simulink model "SpaceXStarshipMotionSimulation"  (R2024b)
settings: Solver=VariableStepAuto  StartTime=0.0  StopTime=60  RelTol=1e-3
values from neighbouring files (symbols this model uses):
  c_p = 55.09    [SpaceX Starship_EarthtoEarth_Sims.m]
  F_t = 74400000    [SpaceX Starship_EarthtoEarth_Sims.m]
  g = 9.81    [SpaceX Starship_EarthtoEarth_Sims.m]
  Ixx = I(1,1)    [SpaceX Starship_EarthtoEarth_Sims.m]
  Izz = I(3,3)    [SpaceX Starship_EarthtoEarth_Sims.m]
  L = 55.74    [SpaceX Starship_EarthtoEarth_Sims.m]
  m_r = 5270000    [SpaceX Starship_EarthtoEarth_Sims.m]
libraries: simulink x9, shared6dof x1, aerolibanim x1
settings Model: Creator=samueljoseph  LastModifiedBy=samueljoseph

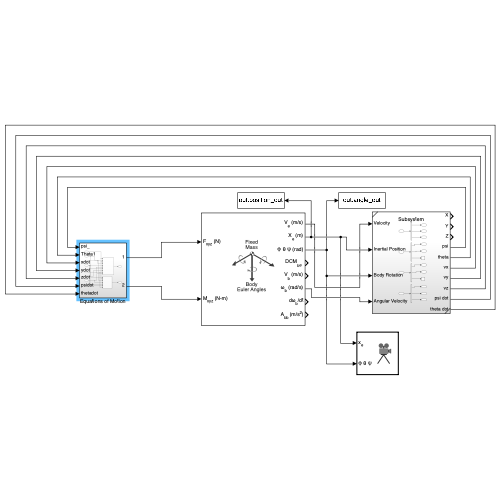
[thumbnail: Simulink's stored preview of the top-level diagram]
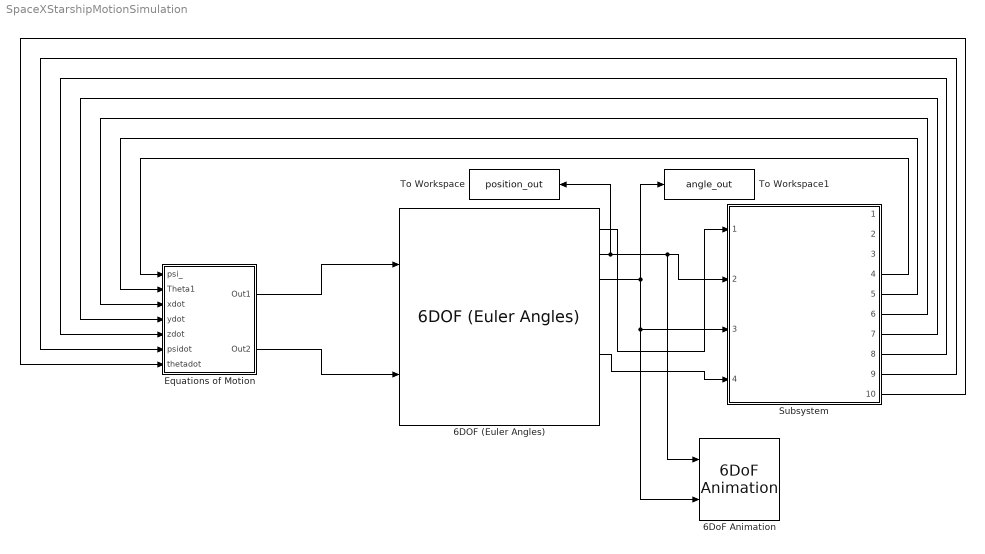
== system SpaceXStarshipMotionSimulation ==
  6DOF (Euler Angles) : shared6dof/6DOF (Euler Angles)  units=Metric (MKS)  mtype=Fixed  rep=Euler Angles  xme_0=[0 0 6371000]  Vm_0=[0 0 0]  eul_0=[pi/4 pi/4 0]  pm_0=[0 0 0]  mass_0=5270000  mass_e=0.5  mass_f=2.0  inertia=[1.9980e9 0 0; 0 1.9980e9 0; 0 0 13069836]  inertia_e=eye(3)  inertia_f=2*eye(3)  k_quat=1.0  vre_flag=on  abi_flag=off  aMode=0  xme_statename=''  Vm_statename=''  eul_statename=''  quat_statename=''  pm_statename=''  mass_statename=''
  6DoF Animation : aerolibanim/6DoF Animation  u1=[0 4000 -2000 2000 -20000 0]  u2=0.1  u3=2000  u4=[4000 0 -5000]  u5=Fly alongside  u6=[5000, 2000, 1000]  u7=45  u8=on
  Equations of Motion : Subsystem
  Subsystem : Subsystem  ReferencedSubsystem=Subsystem
  To Workspace : ToWorkspace  VariableName=position_out  SaveFormat=Timeseries  SampleTime=-1
  To Workspace1 : ToWorkspace  VariableName=angle_out  SaveFormat=Timeseries  SampleTime=-1
  wires:
  6DOF (Euler Angles)/6 -> Subsystem/4
  6DOF (Euler Angles)/2 -> 6DoF Animation/1, Subsystem/2, To Workspace/1
  6DOF (Euler Angles)/3 -> 6DoF Animation/2, Subsystem/3, To Workspace1/1
  6DOF (Euler Angles)/1 -> Subsystem/1
  Subsystem/4 -> Equations of Motion/1(psi_)
  Subsystem/5 -> Equations of Motion/2(Theta1)
  Subsystem/6 -> Equations of Motion/3(xdot)
  Subsystem/7 -> Equations of Motion/4(ydot)
  Subsystem/8 -> Equations of Motion/5(zdot)
  Subsystem/9 -> Equations of Motion/6(psidot)
  Subsystem/10 -> Equations of Motion/7(thetadot)
  Equations of Motion/1(Out1) -> 6DOF (Euler Angles)/1
  Equations of Motion/2(Out2) -> 6DOF (Euler Angles)/2

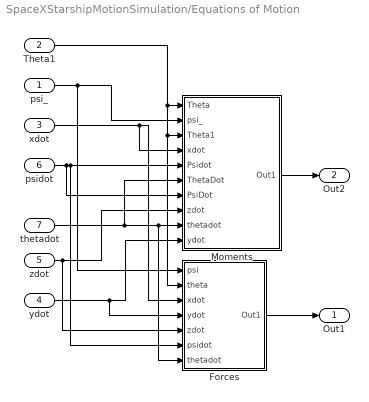
== system SpaceXStarshipMotionSimulation/Equations of Motion ==
  psi_ : Inport
  Theta1 : Inport  Port=2
  xdot : Inport  Port=3
  ydot : Inport  Port=4
  zdot : Inport  Port=5
  psidot : Inport  Port=6
  thetadot : Inport  Port=7
  Forces : Subsystem
  Moments : Subsystem
  Out1 : Outport
  Out2 : Outport  Port=2
  wires:
  Forces/1(Out1) -> Out1/1
  ydot/1 -> Moments/10(ydot), Forces/4(ydot)
  zdot/1 -> Moments/8(zdot), Forces/5(zdot)
  thetadot/1 -> Forces/7(thetadot), Moments/9(thetadot), Moments/6(ThetaDot)
  psidot/1 -> Moments/5(Psidot), Forces/6(psidot), Moments/7(PsiDot)
  xdot/1 -> Moments/4(xdot), Forces/3(xdot)
  Moments/1(Out1) -> Out2/1
  psi_/1 -> Moments/2(psi_), Forces/1(psi)
  Theta1/1 -> Forces/2(theta), Moments/3(Theta1), Moments/1(Theta)

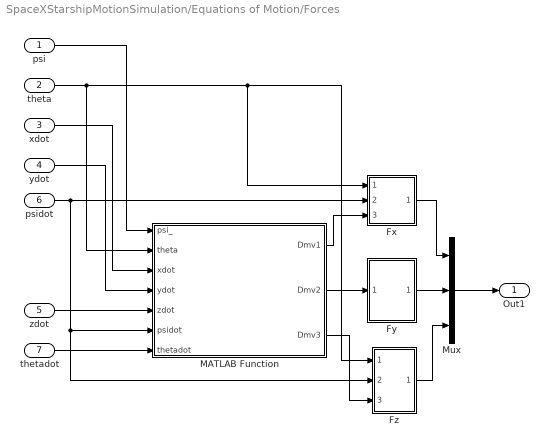
== system SpaceXStarshipMotionSimulation/Equations of Motion/Forces ==
  psi : Inport
  theta : Inport  Port=2
  xdot : Inport  Port=3
  ydot : Inport  Port=4
  zdot : Inport  Port=5
  psidot : Inport  Port=6
  thetadot : Inport  Port=7
  Fx : Subsystem
  Fy : Subsystem
  Fz : Subsystem
  MATLAB Function : MATLAB Function  TreatAsAtomicUnit=on
  Mux : Mux  Inputs=3
  Out1 : Outport
  wires:
  Mux/1 -> Out1/1
  Fz/1(Out1) -> Mux/3
  Fy/1(Out1) -> Mux/2
  Fx/1(Out1) -> Mux/1
  xdot/1 -> MATLAB Function/3(xdot)
  MATLAB Function/3(Dmv3) -> Fz/3(Dmv3)
  psidot/1 -> MATLAB Function/6(psidot), Fz/2(psidot), Fx/2(psidot)
  MATLAB Function/1(Dmv1) -> Fx/3(Dmv1)
  thetadot/1 -> MATLAB Function/7(thetadot)
  ydot/1 -> MATLAB Function/4(ydot)
  MATLAB Function/2(Dmv2) -> Fy/1(Dmv2)
  theta/1 -> MATLAB Function/2(theta), Fz/1(theta), Fx/1(theta)
  zdot/1 -> MATLAB Function/5(zdot)
  psi/1 -> MATLAB Function/1(psi_)

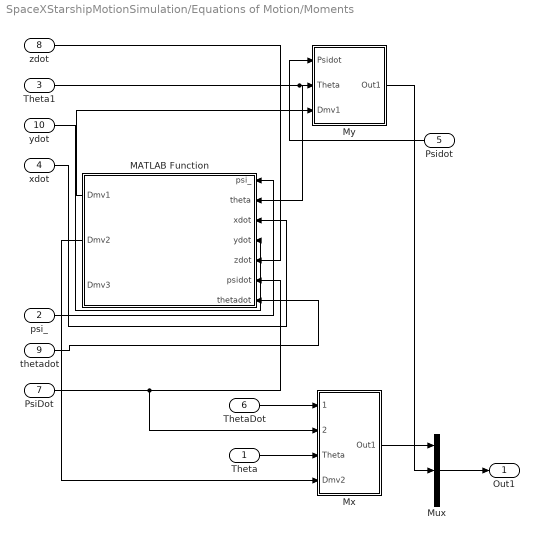
== system SpaceXStarshipMotionSimulation/Equations of Motion/Moments ==
  Theta : Inport
  psi_ : Inport  Port=2
  Theta1 : Inport  Port=3
  xdot : Inport  Port=4
  Psidot : Inport  Port=5
  ThetaDot : Inport  Port=6
  PsiDot : Inport  Port=7
  zdot : Inport  Port=8
  thetadot : Inport  Port=9
  ydot : Inport  Port=10
  MATLAB Function : MATLAB Function  TreatAsAtomicUnit=on
  Mux : Mux  Inputs=3
  Mx : Subsystem
  My : Subsystem
  Out1 : Outport
  wires:
  Psidot/1 -> My/1(Psidot)
  Mx/1(Out1) -> Mux/1
  My/1(Out1) -> Mux/2
  ThetaDot/1 -> Mx/1(ThetaDot)
  MATLAB Function/1(Dmv1) -> My/3(Dmv1)
  Theta/1 -> Mx/3(Theta)
  MATLAB Function/2(Dmv2) -> Mx/4(Dmv2)
  PsiDot/1 -> Mx/2(PsiDot), MATLAB Function/6(psidot)
  thetadot/1 -> MATLAB Function/7(thetadot)
  psi_/1 -> MATLAB Function/1(psi_)
  xdot/1 -> MATLAB Function/3(xdot)
  Mux/1 -> Out1/1
  zdot/1 -> MATLAB Function/5(zdot)
  ydot/1 -> MATLAB Function/4(ydot)
  Theta1/1 -> My/2(Theta), MATLAB Function/2(theta)

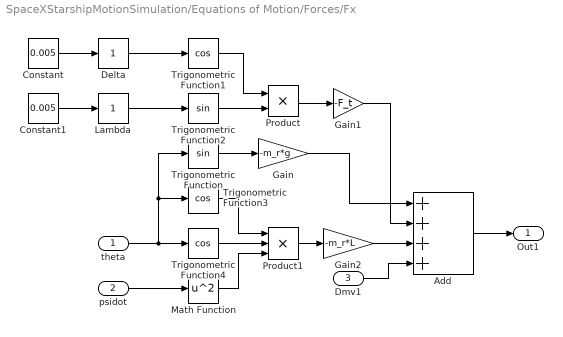
== system SpaceXStarshipMotionSimulation/Equations of Motion/Forces/Fx ==
  theta : Inport
  psidot : Inport  Port=2
  Dmv1 : Inport  Port=3
  Add : Sum  Inputs=++++
  Constant : Constant  Value=0.005
  Constant1 : Constant  Value=0.005
  Delta : simulink/Math Operations/Slider Gain  gain=1  low=0  high=2
  Gain : Gain  Gain=-m_r*g
  Gain1 : Gain  Gain=-F_t
  Gain2 : Gain  Gain=-m_r*L
  Lambda : simulink/Math Operations/Slider Gain  gain=1  low=0  high=2
  Math Function : Math  Operator=square
  Product : Product
  Product1 : Product  Inputs=3
  Trigonometric Function : Trigonometry
  Trigonometric Function1 : Trigonometry  Operator=cos
  Trigonometric Function2 : Trigonometry
  Trigonometric Function3 : Trigonometry  Operator=cos
  Trigonometric Function4 : Trigonometry  Operator=cos
  Out1 : Outport
  wires:
  Dmv1/1 -> Add/4
  Product1/1 -> Gain2/1
  Gain/1 -> Add/1
  Math Function/1 -> Product1/3
  Trigonometric Function4/1 -> Product1/2
  Trigonometric Function3/1 -> Product1/1
  Constant1/1 -> Lambda/1
  Trigonometric Function1/1 -> Product/1
  theta/1 -> Trigonometric Function/1, Trigonometric Function3/1, Trigonometric Function4/1
  Add/1 -> Out1/1
  Gain1/1 -> Add/2
  Trigonometric Function/1 -> Gain/1
  Product/1 -> Gain1/1
  Lambda/1 -> Trigonometric Function2/1
  Delta/1 -> Trigonometric Function1/1
  Trigonometric Function2/1 -> Product/2
  Gain2/1 -> Add/3
  psidot/1 -> Math Function/1
  Constant/1 -> Delta/1

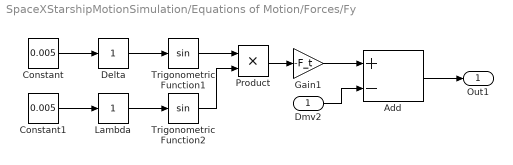
== system SpaceXStarshipMotionSimulation/Equations of Motion/Forces/Fy ==
  Dmv2 : Inport
  Add : Sum  Inputs=+-
  Constant : Constant  Value=0.005
  Constant1 : Constant  Value=0.005
  Delta : simulink/Math Operations/Slider Gain  gain=1  low=0  high=2
  Gain1 : Gain  Gain=-F_t
  Lambda : simulink/Math Operations/Slider Gain  gain=1  low=0  high=2
  Product : Product
  Trigonometric Function1 : Trigonometry
  Trigonometric Function2 : Trigonometry
  Out1 : Outport
  wires:
  Add/1 -> Out1/1
  Product/1 -> Gain1/1
  Gain1/1 -> Add/1
  Trigonometric Function2/1 -> Product/2
  Dmv2/1 -> Add/2
  Trigonometric Function1/1 -> Product/1
  Delta/1 -> Trigonometric Function1/1
  Constant1/1 -> Lambda/1
  Lambda/1 -> Trigonometric Function2/1
  Constant/1 -> Delta/1

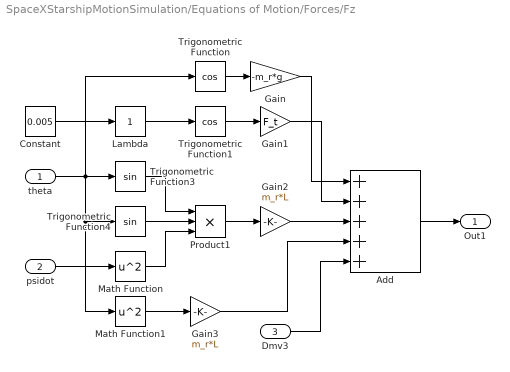
== system SpaceXStarshipMotionSimulation/Equations of Motion/Forces/Fz ==
  theta : Inport
  psidot : Inport  Port=2
  Dmv3 : Inport  Port=3
  Add : Sum  Inputs=+++++
  Constant : Constant  Value=0.005
  Gain : Gain  Gain=-m_r*g
  Gain1 : Gain  Gain=F_t
  Gain2 : Gain  Gain=m_r*L
  Gain3 : Gain  Gain=m_r*L
  Lambda : simulink/Math Operations/Slider Gain  gain=1  low=0  high=2
  Math Function : Math  Operator=square
  Math Function1 : Math  Operator=square
  Product1 : Product  Inputs=3
  Trigonometric Function : Trigonometry  Operator=cos
  Trigonometric Function1 : Trigonometry  Operator=cos
  Trigonometric Function3 : Trigonometry
  Trigonometric Function4 : Trigonometry
  Out1 : Outport
  wires:
  Dmv3/1 -> Add/5
  Gain1/1 -> Add/2
  Gain/1 -> Add/1
  Product1/1 -> Gain2/1
  Trigonometric Function1/1 -> Gain1/1
  Trigonometric Function/1 -> Gain/1
  Math Function1/1 -> Gain3/1
  Math Function/1 -> Product1/3
  Gain3/1 -> Add/4
  Trigonometric Function4/1 -> Product1/2
  Trigonometric Function3/1 -> Product1/1
  Add/1 -> Out1/1
  Lambda/1 -> Trigonometric Function1/1
  theta/1 -> Trigonometric Function/1, Trigonometric Function4/1, Math Function1/1, Trigonometric Function3/1
  psidot/1 -> Math Function/1
  Gain2/1 -> Add/3
  Constant/1 -> Lambda/1

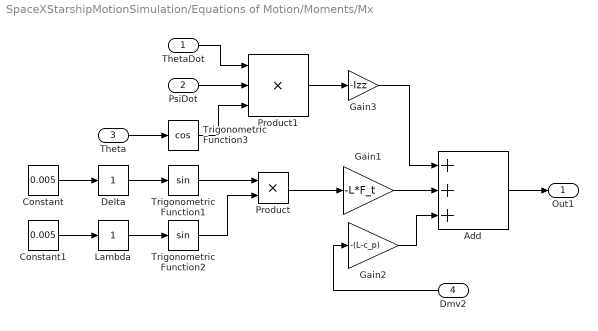
== system SpaceXStarshipMotionSimulation/Equations of Motion/Moments/Mx ==
  ThetaDot : Inport
  PsiDot : Inport  Port=2
  Theta : Inport  Port=3
  Dmv2 : Inport  Port=4
  Add : Sum  Inputs=+++
  Constant : Constant  Value=0.005
  Constant1 : Constant  Value=0.005
  Delta : simulink/Math Operations/Slider Gain  gain=1  low=0  high=2
  Gain1 : Gain  Gain=-L*F_t
  Gain2 : Gain  Gain=-(L-c_p)
  Gain3 : Gain  Gain=-Izz
  Lambda : simulink/Math Operations/Slider Gain  gain=1  low=0  high=2
  Product : Product
  Product1 : Product  Inputs=3
  Trigonometric Function1 : Trigonometry
  Trigonometric Function2 : Trigonometry
  Trigonometric Function3 : Trigonometry  Operator=cos
  Out1 : Outport
  wires:
  Product/1 -> Gain1/1
  Gain1/1 -> Add/2
  PsiDot/1 -> Product1/2
  Product1/1 -> Gain3/1
  Trigonometric Function2/1 -> Product/2
  Dmv2/1 -> Gain2/1
  Trigonometric Function1/1 -> Product/1
  Trigonometric Function3/1 -> Product1/3
  Gain3/1 -> Add/1
  ThetaDot/1 -> Product1/1
  Lambda/1 -> Trigonometric Function2/1
  Delta/1 -> Trigonometric Function1/1
  Theta/1 -> Trigonometric Function3/1
  Add/1 -> Out1/1
  Constant1/1 -> Lambda/1
  Constant/1 -> Delta/1
  Gain2/1 -> Add/3

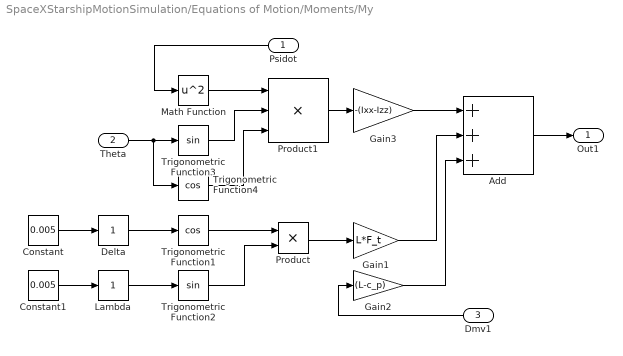
== system SpaceXStarshipMotionSimulation/Equations of Motion/Moments/My ==
  Psidot : Inport
  Theta : Inport  Port=2
  Dmv1 : Inport  Port=3
  Add : Sum  Inputs=+++
  Constant : Constant  Value=0.005
  Constant1 : Constant  Value=0.005
  Delta : simulink/Math Operations/Slider Gain  gain=1  low=0  high=2
  Gain1 : Gain  Gain=L*F_t
  Gain2 : Gain  Gain=(L-c_p)
  Gain3 : Gain  Gain=-(Ixx-Izz)
  Lambda : simulink/Math Operations/Slider Gain  gain=1  low=0  high=2
  Math Function : Math  Operator=square
  Product : Product
  Product1 : Product  Inputs=3
  Trigonometric Function1 : Trigonometry  Operator=cos
  Trigonometric Function2 : Trigonometry
  Trigonometric Function3 : Trigonometry
  Trigonometric Function4 : Trigonometry  Operator=cos
  Out1 : Outport
  wires:
  Add/1 -> Out1/1
  Gain1/1 -> Add/2
  Gain3/1 -> Add/1
  Dmv1/1 -> Gain2/1
  Product/1 -> Gain1/1
  Trigonometric Function2/1 -> Product/2
  Trigonometric Function4/1 -> Product1/3
  Trigonometric Function1/1 -> Product/1
  Math Function/1 -> Product1/1
  Constant/1 -> Delta/1
  Product1/1 -> Gain3/1
  Lambda/1 -> Trigonometric Function2/1
  Constant1/1 -> Lambda/1
  Theta/1 -> Trigonometric Function4/1, Trigonometric Function3/1
  Psidot/1 -> Math Function/1
  Trigonometric Function3/1 -> Product1/2
  Delta/1 -> Trigonometric Function1/1
  Gain2/1 -> Add/3

== matlab function SpaceXStarshipMotionSimulation/Equations of Motion/Moments/MATLAB Function ==
  data: psi_ input; theta input; xdot input; Dmv1 output; ydot input; zdot input; psidot input; thetadot input; Dmv2 output; Dmv3 output
function [Dmv1, Dmv2, Dmv3] = drag(psi_, theta,xdot, ydot, zdot, psidot, thetadot)
L = 55.74; 
CD = 0.6;                        % Coefficient of Drag
A = 63.61;                       % Frontal Nose Area for Drag (m^2)
rho = 1.225;
D_const = (0.5) * CD * rho * A;  % Drag Constant 


phi = psi_;

vx = xdot*cos(phi)*cos(theta) + ydot*sin(phi)*cos(theta) + zdot*sin(theta) + L*thetadot;
vy = ydot*cos(phi) - psidot*L*sin(theta);
vz = xdot*sin(phi)*sin(theta) + zdot*cos(theta);

v_mag = sqrt(vx^2 + vy^2 + vz^2) + 1e-6;
D_mag = D_const * (vx^2 + vy^2 + vz^2);

Dmv1 = D_mag * (vx / v_mag);
Dmv2 = D_mag * (vy / v_mag);
Dmv3 = D_mag * (vz / v_mag);
end

== matlab function SpaceXStarshipMotionSimulation/Equations of Motion/Forces/MATLAB Function ==
  data: psi_ input; theta input; xdot input; Dmv1 output; ydot input; zdot input; psidot input; thetadot input; Dmv2 output; Dmv3 output
function [Dmv1, Dmv2, Dmv3] = drag(psi_, theta,xdot, ydot, zdot, psidot, thetadot)
L = 55.74; 
CD = 0.6;                        % Coefficient of Drag
A = 63.61;                       % Frontal Nose Area for Drag (m^2)
rho = 1.225;
D_const = (0.5) * CD * rho * A;  % Drag Constant 

phi = psi_;
vx = xdot*cos(phi)*cos(theta) + ydot*sin(phi)*cos(theta) + zdot*sin(theta) + L*thetadot;
vy = ydot*cos(phi) - psidot*L*sin(theta);
vz = xdot*sin(phi)*sin(theta) + zdot*cos(theta);

v_mag = sqrt(vx^2 + vy^2 + vz^2) + 1e-6;
D_mag = D_const * (vx^2 + vy^2 + vz^2);

Dmv1 = D_mag * (vx / v_mag);
Dmv2 = D_mag * (vy / v_mag);
Dmv3 = D_mag * (vz / v_mag);
end
